simulink model "A2_adaptive_cruise_control"  (R2023b)
settings: Solver=FixedStepAuto  StartTime=0.0  StopTime=inf  RelTol=1e-3
libraries: dspswit3 x1, Pynq_functions x1, slpidlib x1
settings Model: Creator=20192363  LastModifiedBy=20230981
settings OptimizationCC: DefaultParameterBehavior=Inlined  EnhancedBackFolding=on  PassReuseOutputArgsAs=Individual arguments  ZeroExternalMemoryAtStartup=off  ZeroInternalMemoryAtStartup=off  OptimizeBlockOrder=speed  DifferentSizesBufferReuse=on  OptimizationCustomize=off  EfficientTunableParamExpr=on
settings DebuggingCC: ParameterTunabilityLossMsg=error
settings SFSimCC: MATLABDynamicMemAlloc=off
settings RTWCC: Description=Embedded Coder  SystemTargetFile=ert.tlc  GenCodeOnly=on  TemplateMakefile=ert_default_tmf
settings CodeAppCC: ForceParamTrailComments=on  IgnoreCustomStorageClasses=off  OperatorAnnotations=on  SimulinkDataObjDesc=on  SFDataObjDesc=on  InsertBlockDesc=on
settings ERTTargetCC: TargetLangStandard=C99 (ISO)  GenerateSampleERTMain=on  SupportNonInlinedSFcns=on  InlinedParameterPlacement=NonHierarchical  ERTCustomFileTemplate=example_file_process.tlc

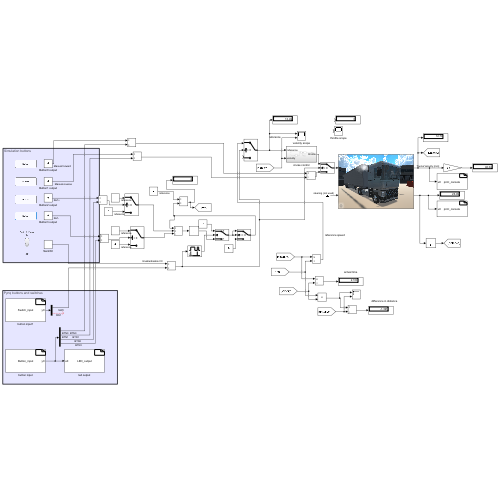
[thumbnail: Simulink's stored preview of the top-level diagram]
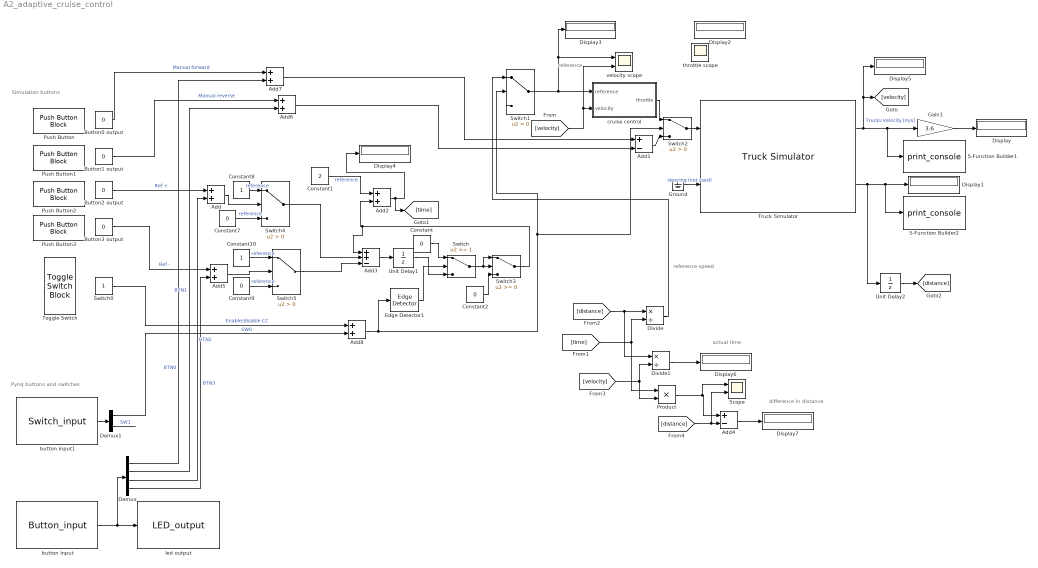
== system A2_adaptive_cruise_control ==
  note: reference speed
  note: reference
  note: Pynq buttons and switches
  note: Simulation buttons
  note: actual time
  note: difference in distance
  Add{,2,5..8} (6 alike) : Sum
  Add1 : Sum  Inputs=+-
  Add3 : Sum  Inputs=++-
  Add4 : Sum  Inputs=+-
  Button0 output : Constant  Value=0
  Button1 output : Constant  Value=0
  Button2 output : Constant  Value=0
  Button3 output : Constant  Value=0
  Constant{,2,7,9} (4 alike) : Constant  Value=0
  Constant1 : Constant  Value=2
  Constant10 : Constant
  Constant8 : Constant
  Demux : Demux
  Demux1 : Demux  Outputs=2
  Display{,1..7} (8 alike) : Display
  Divide : Product  Inputs=*/
  Divide1 : Product  Inputs=*/
  Edge Detector1 : dspswit3/Edge Detector  InputProcessing=Columns as channels (frame based)
  Gain1 : Gain  Gain=3.6
  Ground : Ground
  Product : Product
  Push Button{,1..3} (4 alike) : PushButtonBlock  OffValue=0.000000
  S-Function Builder1 : S-Function  FunctionName=print_console  SFunctionModules=print_console_wrapper.c  SFunctionDeploymentMode=off  EnableBusSupport=off  mask(S-Function Builder){}
      mask help: Simulink:masks:SFunctionBuilder_MD
      mask init:
      | val = [[.9  0.75 0.75 1 1 .9 .9 1]',[1 1 0.75 0.75 .9 .9 1 .9]'];try , sys = get_param(gcb,'SfunBuilderFcnName');if isempty(sys), sys = get_param(gcb,'FunctionName'); end,catch, sys = get_param(gcb,'FunctionName'); end
      settings: CopyFcn=set_param(gcbh,'LinkStatus','none')  OpenFcn=sfunctionwizard(gcbh)
      mask Display:
      | plot(val(:,1),val(:,2))
      | disp(sys)
      | port_label('input',1,'u0')
  S-Function Builder2 : S-Function  FunctionName=print_console  SFunctionModules=print_console_wrapper.c  SFunctionDeploymentMode=off  EnableBusSupport=off  mask(S-Function Builder){}
      mask help: Simulink:masks:SFunctionBuilder_MD
      mask init: same as A2_adaptive_cruise_control/S-Function Builder1
      settings: CopyFcn=set_param(gcbh,'LinkStatus','none')  OpenFcn=sfunctionwizard(gcbh)
      mask Display:
      | plot(val(:,1),val(:,2))
      | disp(sys)
      | port_label('input',1,'u0')
  Scope : Scope  NumInputPorts=2
  Switch : Switch  Threshold=1  SaturateOnIntegerOverflow=off  InputSameDT=off
  Switch0 : Constant
  Switch{1..2,4..5} (4 alike) : Switch  Criteria=u2 > Threshold  SaturateOnIntegerOverflow=off  InputSameDT=off
  Switch3 : Switch  SaturateOnIntegerOverflow=off  InputSameDT=off
  Toggle Switch : ToggleSwitchBlock
      settings: Values={{'Off', 'On'}, [0 1]}
  Truck Simulator : Pynq_functions/Truck Simulator
      link override UDP_pynq: FunctionName=UDP_pynq  SFunctionModules=UDP_pynq_wrapper.c
  Unit Delay1 : UnitDelay  SampleTime=-1  HasFrameUpgradeWarning=on
  Unit Delay2 : UnitDelay  SampleTime=-1  HasFrameUpgradeWarning=on
  button input : S-Function  FunctionName=Button_input  SFunctionModules=Button_input_wrapper.c  SFunctionDeploymentMode=off  EnableBusSupport=off  mask(S-Function Builder){}
      mask help: Simulink:masks:SFunctionBuilder_MD
      mask init: same as A2_adaptive_cruise_control/S-Function Builder1
      settings: CopyFcn=set_param(gcbh,'LinkStatus','none')  OpenFcn=sfunctionwizard(gcbh)
      mask Display: plot(val(:,1),val(:,2)),disp(sys),port_label('output',1,'y0')
  button input1 : S-Function  FunctionName=Switch_input  SFunctionModules=Switch_input_wrapper.c  SFunctionDeploymentMode=off  EnableBusSupport=off  mask(S-Function Builder){}
      mask help: Simulink:masks:SFunctionBuilder_MD
      mask init: same as A2_adaptive_cruise_control/S-Function Builder1
      settings: CopyFcn=set_param(gcbh,'LinkStatus','none')  OpenFcn=sfunctionwizard(gcbh)
      mask Display:
      | plot(val(:,1),val(:,2))
      | disp(sys)
      | port_label('output',1,'y0')
  cruise control : Subsystem
  led output : S-Function  FunctionName=LED_output  SFunctionModules=LED_output_wrapper.c  SFunctionDeploymentMode=off  EnableBusSupport=off  mask(S-Function Builder){}
      mask help: Simulink:masks:SFunctionBuilder_MD
      mask init: same as A2_adaptive_cruise_control/S-Function Builder1
      settings: CopyFcn=set_param(gcbh,'LinkStatus','none')  OpenFcn=sfunctionwizard(gcbh)
      mask Display: plot(val(:,1),val(:,2)),disp(sys),port_label('input',1,'u0')
  throttle scope : Scope
  velocity scope : Scope  NumInputPorts=2
  wires:
  Truck Simulator/1 -> [velocity], Display5/1, S-Function Builder1/1, Gain1/1  "Trucks Velocity [m/s]"
  button input/1 -> Demux/1, led output/1
  Truck Simulator/2 -> Unit Delay2/1, Display1/1, S-Function Builder2/1
  Ground/1 -> Truck Simulator/2  "steering (not used)"
  button input1/1 -> Demux1/1
  Demux1/1 -> Add8/2  "SW0"
  Demux1/2 -> ?  "SW1"
  Demux/3 -> Add/2  "BTN2"
  Demux/4 -> Add5/2  "BTN3"
  Switch0/1 -> Add8/1  "Enable/disable CC"
  [velocity] -> cruise control/2(velocity), velocity scope/2
  Switch1/1 -> cruise control/1(reference), velocity scope/1, Display3/1
  Gain1/1 -> Display/1
  Constant10/1 -> Switch5/1  "reference"
  Switch4/1 -> Add3/2
  Constant7/1 -> Switch4/3  "reference"
  Constant1/1 -> Add2/1  "reference"
  Constant9/1 -> Switch5/3  "reference"
  Constant8/1 -> Switch4/1  "reference"
  Add3/1 -> Unit Delay1/1
  Switch5/1 -> Add3/3
  Button2 output/1 -> Add/1  "Ref +"
  Button3 output/1 -> Add5/1  "Ref -"
  Add2/1 -> [time], Display4/1
  [distance] -> Divide/1, Divide1/1
  [time] -> Divide/2, Product/1
  Divide/1 -> Switch1/1
  Unit Delay2/1 -> [distance]
  [velocity] -> Divide1/2, Product/2
  Divide1/1 -> Display6/1
  [distance] -> Scope/2, Add4/2
  Product/1 -> Scope/1, Add4/1
  Add4/1 -> Display7/1
  Button0 output/1 -> Add7/1  "Manual forward"
  Button1 output/1 -> Add6/1  "Manual reverse"
  Add6/1 -> Add1/2
  Add7/1 -> Add1/1
  Demux/1 -> Add7/2  "BTN0"
  Demux/2 -> Add6/2  "BTN1"
  Switch2/1 -> Truck Simulator/1
  Add/1 -> Switch4/2
  Add5/1 -> Switch5/2
  Add8/1 -> Switch1/2, Switch2/2, Edge Detector1/1
  Edge Detector1/1 -> Switch/2
  Constant/1 -> Switch/1
  Unit Delay1/1 -> Switch/3
  cruise control/1(throttle) -> Switch2/1
  Switch/1 -> Switch3/1, Switch3/2
  Constant2/1 -> Switch3/3
  Switch3/1 -> Add3/1, Add2/2
  Add1/1 -> Switch2/3

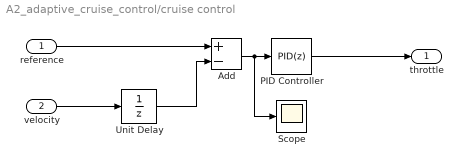
== system A2_adaptive_cruise_control/cruise control ==
  reference : Inport
  velocity : Inport  Port=2
  Add : Sum  Inputs=+-
  PID Controller : slpidlib/PID Controller  Controller=PID  Form=Parallel  TimeDomain=Discrete-time  UseExternalTs=off  SampleTime=0.1  IntegratorMethod=Forward Euler  FilterMethod=Forward Euler  ControllerParametersSource=internal  P=0.5  I=0  UseKiTs=off  D=0  N=100  UseFilter=on  TunerSelectOption=Transfer Function Based (PID Tuner App)  InitialConditionSource=internal  InitialConditionForIntegrator=0  InitialConditionForFilter=0  DifferentiatorICPrevScaledInput=0  ExternalReset=none  TrackingMode=off  Kt=1  LimitOutput=off  SatLimitsSource=internal  UpperSaturationLimit=inf  LowerSaturationLimit=-inf  LinearizeAsGain=on  AntiWindupMode=none  Kb=1  LimitIntegrator=off  UpperIntegratorSaturationLimit=inf  LowerIntegratorSaturationLimit=-inf  POutMin=[]  POutMax=[]  IOutMin=[]  IOutMax=[]  DOutMin=[]  DOutMax=[]  NOutMin=[]  NOutMax=[]  SumOutMin=[]  SumOutMax=[]  SaturationOutMin=[]  SaturationOutMax=[]  PParamMin=[]  PParamMax=[]  IParamMin=[]  IParamMax=[]  DParamMin=[]  DParamMax=[]  NParamMin=[]  NParamMax=[]  KbParamMin=[]  KbParamMax=[]  KtParamMin=[]  KtParamMax=[]  KbOutMin=[]  KbOutMax=[]  KtOutMin=[]  KtOutMax=[]  IntegratorOutMin=[]  IntegratorOutMax=[]  FilterOutMin=[]  FilterOutMax=[]  SumI1OutMin=[]  SumI1OutMax=[]  SumI2OutMin=[]  SumI2OutMax=[]  SumI3OutMin=[]  SumI3OutMax=[]  SumI4OutMin=[]  SumI4OutMax=[]  SumDOutMin=[]  SumDOutMax=[]  DifferentiatorOutMin=[]  DifferentiatorOutMax=[]  FilterDiffOutCoefMin=[]  FilterDiffOutCoefMax=[]  ReciprocalOutMin=[]  ReciprocalOutMax=[]  SumDenOutMin=[]  SumDenOutMax=[]  SumNumOutMin=[]  SumNumOutMax=[]  DivideOutMin=[]  DivideOutMax=[]  UdiffTsProdOutMin=[]  UdiffTsProdOutMax=[]  NTsProdOutMin=[]  NTsProdOutMax=[]  UintegralTsProdOutMin=[]  UintegralTsProdOutMax=[]  UngainTsProdOutMin=[]  UngainTsProdOutMax=[]  ClampingZeroOutDataTypeStr=Inherit: Inherit via back propagation  ClampingZeroOutMin=[]  ClampingZeroOutMax=[]  FilterDenConstantOutDataTypeStr=Inherit: Inherit via back propagation  FilterDenConstantOutMin=[]  FilterDenConstantOutMax=[]  PCopyOutDataTypeStr=Inherit: Inherit via back propagation  PCopyOutMin=[]  PCopyOutMax=[]  NCopyOutDataTypeStr=Inherit: Inherit via back propagation  NCopyOutMin=[]  NCopyOutMax=[]  IntegratorContinuousStateAttributes=''  IntegratorStateMustResolveToSignalObject=off  IntegratorRTWStateStorageClass=Auto  FilterContinuousStateAttributes=''  FilterStateMustResolveToSignalObject=off  FilterRTWStateStorageClass=Auto  ParallelPVariant=InternalParameters  IdealPVariant=Disabled  IVariant=InternalParameters  DVariant=InternalParameters  IntegratorVariant=Discrete  SatVariant=Disabled  AWVariant=Passthrough  PCopyVariant=Disabled  TRVariant=Disabled  FdbkBlocksVariant=Forward  IdealPFdbkVariant=Disabled  SatFdbkVariant=Disabled  DerivativeFilterVariant=ForwardEulerFilter  NVariant=InternalParameters  NCopyVariant=Disabled  FilterICVariant=InternalICsFilter  IntegratorICVariant=InternalICs  ExternalResetVariant=Disabled  TRSumVariant=Passthrough  SumFdbkVariant=Disabled  SumVariant=Sum_PID  TsampFilterVariant=InternalTs  TsampNgainVariant=Passthrough  TsampIntegralVariant=Disabled_SignalSpec  ExternalSaturationOutDataTypeStr=Inherit: Same as second input
  Scope : Scope
  Unit Delay : UnitDelay  SampleTime=-1  HasFrameUpgradeWarning=on
  throttle : Outport
  wires:
  velocity/1 -> Unit Delay/1
  PID Controller/1 -> throttle/1
  Add/1 -> Scope/1, PID Controller/1
  reference/1 -> Add/1
  Unit Delay/1 -> Add/2
